simulink subsystem "comparator"  (R2025b)
settings: Solver=VariableStepAuto  StartTime=0.0  StopTime=10.0  RelTol=1e-3
libraries: simulink x1
settings Model: Creator=brianli  LastModifiedBy=brianli

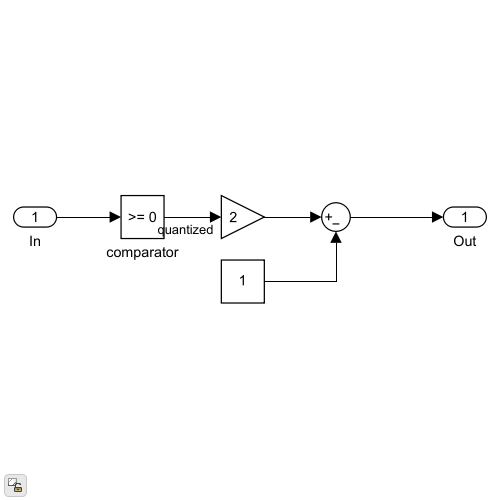
[thumbnail: Simulink's stored preview of the top-level diagram]
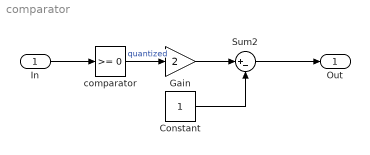
== system comparator ==
  In : Inport
  Constant : Constant
  Gain : Gain  Gain=2  OutDataTypeStr=double
  Sum2 : Sum  Inputs=|+-
  comparator : simulink/Logic and Bit Operations/Compare To Zero  relop=>=  OutDataTypeStr=boolean
      settings: LibrarySourceBlock=|
      | simulink/Quick Insert/Logic and Bit
      | Operations/IsNonNegative
  Out : Outport
  wires:
  comparator/1 -> Gain/1  "quantized"
  Gain/1 -> Sum2/1
  Constant/1 -> Sum2/2
  In/1 -> comparator/1
  Sum2/1 -> Out/1
